simulink model "kalmanssim"  (R2018a)
settings: Solver=VariableStepAuto  StartTime=0.0  StopTime=10.0  RelTol=1e-3
settings Model: Creator=GRENTOR  LastModifiedBy=GRENTOR

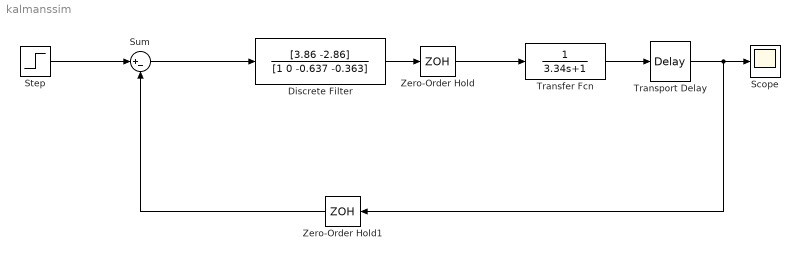
== system kalmanssim ==
  Discrete Filter : DiscreteFilter  Numerator=[3.86 -2.86]  Denominator=[1 0 -0.637 -0.363]  SampleTime=1
  Scope : Scope
  Step : Step  SampleTime=1
  Sum : Sum  Inputs=|+-
  Transfer Fcn : TransferFcn  Denominator=[3.34 1]
  Transport Delay : TransportDelay  DelayTime=1.40  PadeOrder=1
  Zero-Order Hold : ZeroOrderHold
  Zero-Order Hold1 : ZeroOrderHold
  wires:
  Step/1 -> Sum/1
  Sum/1 -> Discrete Filter/1
  Discrete Filter/1 -> Zero-Order Hold/1
  Zero-Order Hold/1 -> Transfer Fcn/1
  Transfer Fcn/1 -> Transport Delay/1
  Transport Delay/1 -> Zero-Order Hold1/1, Scope/1
  Zero-Order Hold1/1 -> Sum/2
